simulink subsystem "Data_Formatter"  (R2023b)
settings: Solver=VariableStepAuto  StartTime=0.0  StopTime=10.0  RelTol=1e-3
settings Model: Creator=victor  LastModifiedBy=victor

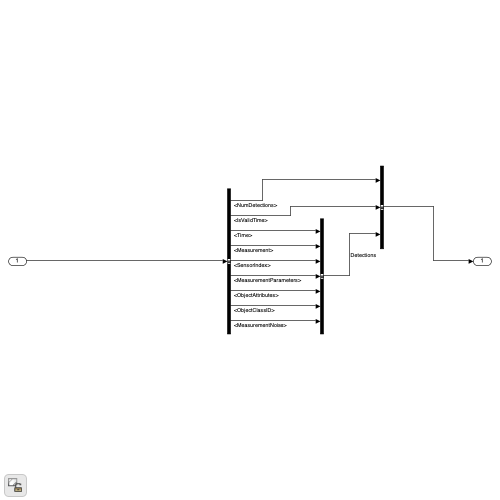
[thumbnail: Simulink's stored preview of the top-level diagram]
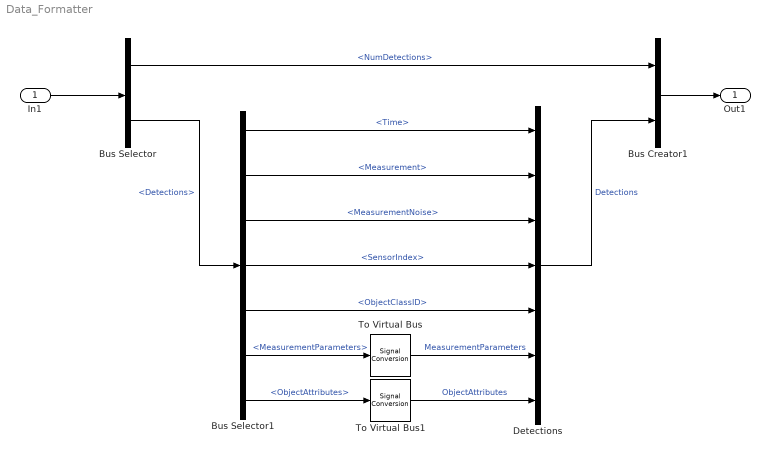
== system Data_Formatter ==
  In1 : Inport
  Bus Creator1 : BusCreator  Inputs=2
  Bus Selector : BusSelector  OutputSignals=NumDetections,Detections
  Bus Selector1 : BusSelector  OutputSignals=Time,Measurement,MeasurementNoise,SensorIndex,ObjectClassID,MeasurementParameters,ObjectAttributes
  Detections : BusCreator  Inputs=7
  To Virtual Bus : SignalConversion  ConversionOutput=Virtual bus  OverrideOpt=off
  To Virtual Bus1 : SignalConversion  ConversionOutput=Virtual bus  OverrideOpt=off
  Out1 : Outport
  wires:
  In1/1 -> Bus Selector/1
  Bus Selector/1 -> Bus Creator1/1  "<NumDetections>"
  Bus Creator1/1 -> Out1/1
  Bus Selector/2 -> Bus Selector1/1  "<Detections>"
  Bus Selector1/1 -> Detections/1  "<Time>"
  Bus Selector1/2 -> Detections/2  "<Measurement>"
  Bus Selector1/6 -> To Virtual Bus/1  "<MeasurementParameters>"
  To Virtual Bus/1 -> Detections/6  "MeasurementParameters"
  Bus Selector1/7 -> To Virtual Bus1/1  "<ObjectAttributes>"
  To Virtual Bus1/1 -> Detections/7  "ObjectAttributes"
  Bus Selector1/5 -> Detections/5  "<ObjectClassID>"
  Bus Selector1/4 -> Detections/4  "<SensorIndex>"
  Bus Selector1/3 -> Detections/3  "<MeasurementNoise>"
  Detections/1 -> Bus Creator1/2  "Detections"
